simulink model "HeatFlowDrive_D"  (Simulink 7.6)
settings: Solver=ode45  StartTime=0.0  StopTime="SimulTime "  RelTol=1e-3
values from neighbouring files (symbols this model uses):
  R = 25    [ParametersHeatFlow_D.m]
  sb = 5.67*(10^-8)    (= 5.67e-08)    [ParametersHeatFlow_D.m]
undefined symbols (not defined in the file or in its folder): Drive, Job, magnitude
libraries: simulink x1
settings Model: Creator=conid  LastModifiedBy=conid

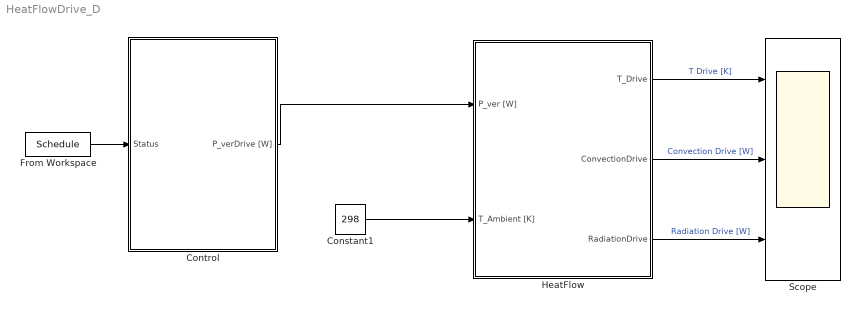
== system HeatFlowDrive_D ==
  Constant1 : Constant  Value=298
  Control : Subsystem  TreatAsAtomicUnit=on  mask{Heat=[0 1 1 1 1], Job=Job}
      mask prompts: Job "Job Struct"
      mask help:
      | Controls the components of the machine:
      |
      | Status:
      |     0. Off
      |     1. Standby
      |     2. Warmup
      |     3. Setting
      |     4. Machining
      |
      | If the status is machining, the job defined as
      |     - Job.time
      |     - Job.omega_dem
      |     - Job.M_dem
      | will be runned, and repeated.
      mask TabNameString: Status,Job
  From Workspace : FromWorkspace  VariableName=Schedule  SampleTime=0  Interpolate=off  OutputAfterFinalValue=Holding final value
  HeatFlow : Subsystem  TreatAsAtomicUnit=on
  Scope : Scope  NumInputPorts=3
      settings: YMin=-5~-5~-5  YMax=5~5~5  SaveName=Scp_HeatFlow
  wires:
  Control/1(P_verDrive [W]) -> HeatFlow/1(P_ver [W])
  Constant1/1 -> HeatFlow/2(T_Ambient [K])
  HeatFlow/1(T_Drive) -> Scope/1  "T Drive [K]"
  HeatFlow/2(ConvectionDrive) -> Scope/2  "Convection Drive [W]"
  HeatFlow/3(RadiationDrive) -> Scope/3  "Radiation Drive [W]"
  From Workspace/1 -> Control/1(Status)

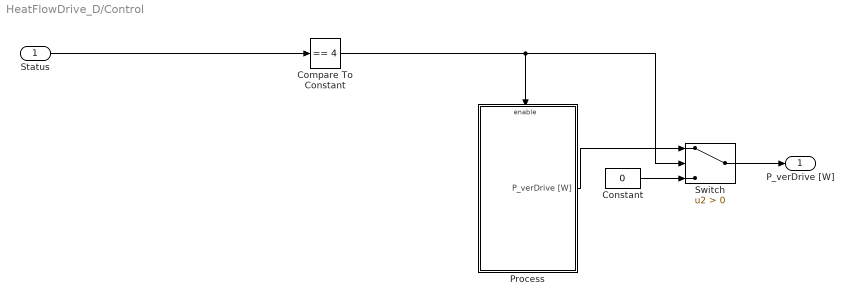
== system HeatFlowDrive_D/Control ==
  Status : Inport
  Compare To Constant : simulink/Logic and Bit Operations/Compare To Constant  SystemSampleTime=-1  relop===  const=4  LogicOutDataTypeMode=uint8
  Constant : Constant  Value=0
  Process : Subsystem  TreatAsAtomicUnit=on
  Switch : Switch  Criteria=u2 > Threshold
  P_verDrive [W] : Outport
  wires:
  Status/1 -> Compare To Constant/1
  Compare To Constant/1 -> Process/Enable, Switch/2
  Process/1(P_verDrive [W]) -> Switch/1
  Constant/1 -> Switch/3
  Switch/1 -> P_verDrive [W]/1

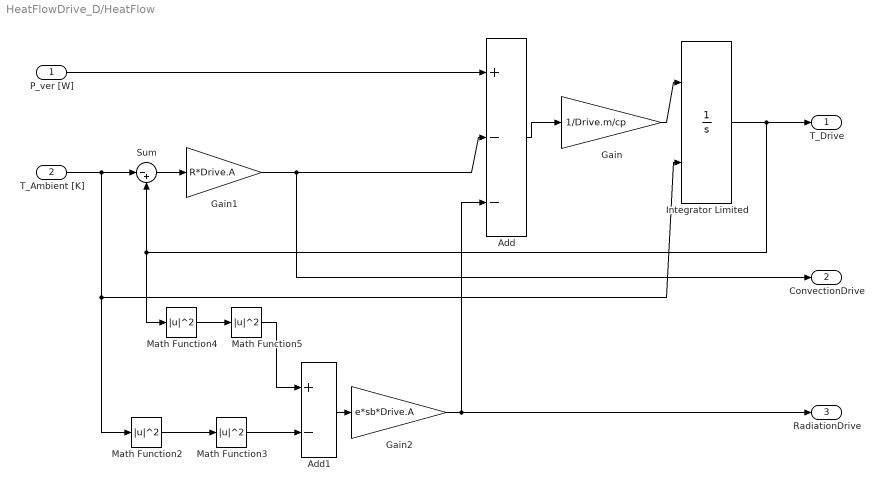
== system HeatFlowDrive_D/HeatFlow ==
  P_ver [W] : Inport
  T_Ambient [K] : Inport  Port=2
  Add : Sum  Inputs=+--
  Add1 : Sum  Inputs=+-
  Gain : Gain  Gain=1/Drive.m/cp
  Gain1 : Gain  Gain=R*Drive.A
  Gain2 : Gain  Gain=e*sb*Drive.A
  Integrator Limited : Integrator  InitialConditionSource=external  LimitOutput=on  ZeroCross=off
  Math Function{2..5} (4 alike) : Math  Operator=magnitude^2  SaturateOnIntegerOverflow=on
  Sum : Sum  Inputs=|-+
  T_Drive : Outport
  ConvectionDrive : Outport  Port=2
  RadiationDrive : Outport  Port=3
  wires:
  P_ver [W]/1 -> Add/1
  T_Ambient [K]/1 -> Sum/1, Integrator Limited/2, Math Function2/1
  Sum/1 -> Gain1/1
  Gain/1 -> Integrator Limited/1
  Gain1/1 -> Add/2, ConvectionDrive/1
  Integrator Limited/1 -> T_Drive/1, Sum/2, Math Function4/1
  Add/1 -> Gain/1
  Gain2/1 -> Add/3, RadiationDrive/1
  Math Function2/1 -> Math Function3/1
  Math Function4/1 -> Math Function5/1
  Math Function5/1 -> Add1/1
  Math Function3/1 -> Add1/2
  Add1/1 -> Gain2/1

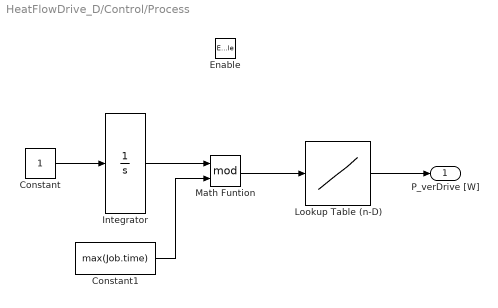
== system HeatFlowDrive_D/Control/Process ==
  Enable : EnablePort
  Constant : Constant
  Constant1 : Constant  Value=max(Job.time)
  Integrator : Integrator
  Lookup Table (n-D) : Lookup_n-D  NumberOfTableDimensions=1  BreakpointsForDimension1=Job.time  Table=Job.P_verDrive  InterpMethod=None - Flat  ExtrapMethod=None - Clip  InputSameDT=on
  Math Funtion : Math  Operator=mod  SaturateOnIntegerOverflow=on
  P_verDrive [W] : Outport
  wires:
  Constant/1 -> Integrator/1
  Integrator/1 -> Math Funtion/1
  Math Funtion/1 -> Lookup Table (n-D)/1
  Lookup Table (n-D)/1 -> P_verDrive [W]/1
  Constant1/1 -> Math Funtion/2
